simulink model "ModeStEnCtrl6s7s"  (R2018b)
settings: Solver=FixedStepDiscrete  StartTime=0.0  StopTime=10.0  FixedStep=0.01  RelTol=1e-3
undefined symbols (not defined in the file or in its folder): BigFour6sStEnCtrl_Cal, BigFourStEnCtrl_Cal, ComfortMdLStEnCtrl_Cal, ComfortMdRStEnCtrl_Cal, EZE5576sStEnCtrl_Cal, EZE557StEnCtrl_Cal, EZQStEnCtrl_Cal, FirstTrig, INTMLStEnCtrl_Cal, INTMRStEnCtrl_Cal, KeSMSuVehicleModelConfig_Val, LugL6sStEnCtrl_Cal, LugL7sStEnCtrl_Cal, LugR6sStEnCtrl_Cal, LugR7sStEnCtrl_Cal, Md27StEnCtrl_Cal, Md28StEnCtrl_Cal, Md30StEnCtrl_Cal, Md31StEnCtrl_Cal, Md32StEnCtrl_Cal, Md53StEnCtrl_Cal, Md57StEnCtrl_Cal, Md58StEnCtrl_Cal, Md58TrgtPos_Set, Md61StEnCtrl_Cal, Md62StEnCtrl_Cal, RecvR4sStEnCtrl_Cal, VIPL557LTStEnCtrl_Cal, VIPL557StEnCtrl_Cal, VIPLExit557StEnCtrl_Cal, VIPLExit557TrgtPos_Set, VIPR557LTStEnCtrl_Cal, VIPR557StEnCtrl_Cal, VIPRExit557StEnCtrl_Cal, VIPRExit557TrgtPos_Set
libraries: simulink x30
(part 2 of 2)

== system ModeStEnCtrl6s7s/ModeStEnCtrl6s7s_Cal_sys/Subsystem/FamlyLStEnCtrl ==
  note: Delete block
  Enable : EnablePort  StatesWhenEnabling=reset
  Constant : Constant  Value=0  OutDataTypeStr=boolean
  Md62StEnCtrl_Cal : FunctionCaller  FunctionPrototype=Md62StEnCtrl_Cal(FirstTrig)  InputArgumentSpecifications=boolean(true)  OutputArgumentSpecifications=<Enter example>
  Unit Delay : UnitDelay  InitialCondition=1  SampleTime=-1  HasFrameUpgradeWarning=on
  wires:
  Unit Delay/1 -> Md62StEnCtrl_Cal/1
  Constant/1 -> Unit Delay/1

== system ModeStEnCtrl6s7s/ModeStEnCtrl6s7s_Cal_sys/Subsystem/FamlyRStEnCtrl ==
  note: Delete block
  Enable : EnablePort  StatesWhenEnabling=reset
  Constant : Constant  Value=0  OutDataTypeStr=boolean
  Md61StEnCtrl_Cal : FunctionCaller  FunctionPrototype=Md61StEnCtrl_Cal(FirstTrig)  InputArgumentSpecifications=boolean(true)  OutputArgumentSpecifications=<Enter example>
  Unit Delay : UnitDelay  InitialCondition=1  SampleTime=-1  HasFrameUpgradeWarning=on
  wires:
  Unit Delay/1 -> Md61StEnCtrl_Cal/1
  Constant/1 -> Unit Delay/1

== system ModeStEnCtrl6s7s/ModeStEnCtrl6s7s_Cal_sys/Subsystem/INTMLStEnCtrl ==
  note: Delete block
  note: Delete block
  Enable : EnablePort
  INTMLStEnCtrl_Cal : FunctionCaller  FunctionPrototype=INTMLStEnCtrl_Cal()  InputArgumentSpecifications=<Enter example>  OutputArgumentSpecifications=<Enter example>

== system ModeStEnCtrl6s7s/ModeStEnCtrl6s7s_Cal_sys/Subsystem/INTMRStEnCtrl ==
  note: Delete block
  note: Delete block
  Enable : EnablePort
  INTMRStEnCtrl_Cal : FunctionCaller  FunctionPrototype=INTMRStEnCtrl_Cal()  InputArgumentSpecifications=<Enter example>  OutputArgumentSpecifications=<Enter example>

== system ModeStEnCtrl6s7s/ModeStEnCtrl6s7s_Cal_sys/Subsystem/Lug6sLStEnCtrl ==
  note: Delete block
  Enable : EnablePort  StatesWhenEnabling=reset
  LugL6sStEnCtrl_Cal : FunctionCaller  FunctionPrototype=LugL6sStEnCtrl_Cal()  InputArgumentSpecifications=<Enter example>  OutputArgumentSpecifications=<Enter example>

== system ModeStEnCtrl6s7s/ModeStEnCtrl6s7s_Cal_sys/Subsystem/Lug6sRStEnCtrl ==
  note: Delete block
  Enable : EnablePort  StatesWhenEnabling=reset
  LugR6sStEnCtrl_Cal : FunctionCaller  FunctionPrototype=LugR6sStEnCtrl_Cal()  InputArgumentSpecifications=<Enter example>  OutputArgumentSpecifications=<Enter example>

== system ModeStEnCtrl6s7s/ModeStEnCtrl6s7s_Cal_sys/Subsystem/Lug7sLStEnCtrl ==
  Enable : EnablePort  StatesWhenEnabling=reset
  Constant : Constant  Value=0  OutDataTypeStr=boolean
  LugL7sStEnCtrl_Cal : FunctionCaller  FunctionPrototype=LugL7sStEnCtrl_Cal(FirstTrig)  InputArgumentSpecifications=boolean(true)  OutputArgumentSpecifications=<Enter example>
  Unit Delay : UnitDelay  InitialCondition=1  SampleTime=-1  HasFrameUpgradeWarning=on
  wires:
  Unit Delay/1 -> LugL7sStEnCtrl_Cal/1
  Constant/1 -> Unit Delay/1

== system ModeStEnCtrl6s7s/ModeStEnCtrl6s7s_Cal_sys/Subsystem/Lug7sRStEnCtrl ==
  Enable : EnablePort  StatesWhenEnabling=reset
  Constant : Constant  Value=0  OutDataTypeStr=boolean
  LugR7sStEnCtrl_Cal : FunctionCaller  FunctionPrototype=LugR7sStEnCtrl_Cal(FirstTrig)  InputArgumentSpecifications=boolean(true)  OutputArgumentSpecifications=<Enter example>
  Unit Delay : UnitDelay  InitialCondition=1  SampleTime=-1  HasFrameUpgradeWarning=on
  wires:
  Unit Delay/1 -> LugR7sStEnCtrl_Cal/1
  Constant/1 -> Unit Delay/1

== system ModeStEnCtrl6s7s/ModeStEnCtrl6s7s_Cal_sys/Subsystem/Md27StEnCtrl ==
  Enable : EnablePort  StatesWhenEnabling=reset
  Constant : Constant  Value=0  OutDataTypeStr=boolean
  Unit Delay : UnitDelay  InitialCondition=1  SampleTime=-1  HasFrameUpgradeWarning=on
  VIPLExit557StEnCtrl_Cal : FunctionCaller  FunctionPrototype=VIPLExit557StEnCtrl_Cal(FirstTrig)  InputArgumentSpecifications=boolean(true)  OutputArgumentSpecifications=<Enter example>
  wires:
  Constant/1 -> Unit Delay/1
  Unit Delay/1 -> VIPLExit557StEnCtrl_Cal/1

== system ModeStEnCtrl6s7s/ModeStEnCtrl6s7s_Cal_sys/Subsystem/Md27StEnCtrl358  ==
  note: Delete block
  Enable : EnablePort  StatesWhenEnabling=reset
  Md27StEnCtrl_Cal : FunctionCaller  FunctionPrototype=Md27StEnCtrl_Cal()  InputArgumentSpecifications=<Enter example>  OutputArgumentSpecifications=<Enter example>

== system ModeStEnCtrl6s7s/ModeStEnCtrl6s7s_Cal_sys/Subsystem/Md28StEnCtrl ==
  Enable : EnablePort  StatesWhenEnabling=reset
  Constant : Constant  Value=0  OutDataTypeStr=boolean
  Unit Delay : UnitDelay  InitialCondition=1  SampleTime=-1  HasFrameUpgradeWarning=on
  VIPRExit557StEnCtrl_Cal : FunctionCaller  FunctionPrototype=VIPRExit557StEnCtrl_Cal(FirstTrig)  InputArgumentSpecifications=boolean(true)  OutputArgumentSpecifications=<Enter example>
  wires:
  Constant/1 -> Unit Delay/1
  Unit Delay/1 -> VIPRExit557StEnCtrl_Cal/1

== system ModeStEnCtrl6s7s/ModeStEnCtrl6s7s_Cal_sys/Subsystem/Md28StEnCtrl358  ==
  note: Delete block
  Enable : EnablePort  StatesWhenEnabling=reset
  Md28StEnCtrl_Cal : FunctionCaller  FunctionPrototype=Md28StEnCtrl_Cal()  InputArgumentSpecifications=<Enter example>  OutputArgumentSpecifications=<Enter example>

== system ModeStEnCtrl6s7s/ModeStEnCtrl6s7s_Cal_sys/Subsystem/Md30StEnCtrl ==
  Enable : EnablePort  StatesWhenEnabling=reset
  Constant : Constant  Value=0  OutDataTypeStr=boolean
  Md30StEnCtrl_Cal : FunctionCaller  FunctionPrototype=Md30StEnCtrl_Cal(FirstTrig)  InputArgumentSpecifications=boolean(true)  OutputArgumentSpecifications=<Enter example>
  Unit Delay : UnitDelay  InitialCondition=1  SampleTime=-1  HasFrameUpgradeWarning=on
  wires:
  Constant/1 -> Unit Delay/1
  Unit Delay/1 -> Md30StEnCtrl_Cal/1

== system ModeStEnCtrl6s7s/ModeStEnCtrl6s7s_Cal_sys/Subsystem/Md31StEnCtrl ==
  Enable : EnablePort  StatesWhenEnabling=reset
  Constant : Constant  Value=0  OutDataTypeStr=boolean
  Md31StEnCtrl_Cal : FunctionCaller  FunctionPrototype=Md31StEnCtrl_Cal(FirstTrig)  InputArgumentSpecifications=boolean(true)  OutputArgumentSpecifications=<Enter example>
  Unit Delay : UnitDelay  InitialCondition=1  SampleTime=-1  HasFrameUpgradeWarning=on
  wires:
  Constant/1 -> Unit Delay/1
  Unit Delay/1 -> Md31StEnCtrl_Cal/1

== system ModeStEnCtrl6s7s/ModeStEnCtrl6s7s_Cal_sys/Subsystem/Md32StEnCtrl ==
  Enable : EnablePort  StatesWhenEnabling=reset
  Constant : Constant  Value=0  OutDataTypeStr=boolean
  Md32StEnCtrl_Cal : FunctionCaller  FunctionPrototype=Md32StEnCtrl_Cal(FirstTrig)  InputArgumentSpecifications=boolean(true)  OutputArgumentSpecifications=<Enter example>
  Unit Delay : UnitDelay  InitialCondition=1  SampleTime=-1  HasFrameUpgradeWarning=on
  wires:
  Constant/1 -> Unit Delay/1
  Unit Delay/1 -> Md32StEnCtrl_Cal/1

== system ModeStEnCtrl6s7s/ModeStEnCtrl6s7s_Cal_sys/Subsystem/Md53StEnCtrl ==
  Enable : EnablePort  StatesWhenEnabling=reset
  Constant : Constant  Value=0  OutDataTypeStr=boolean
  Md53StEnCtrl_Cal : FunctionCaller  FunctionPrototype=Md53StEnCtrl_Cal(FirstTrig)  InputArgumentSpecifications=boolean(true)  OutputArgumentSpecifications=<Enter example>
  Unit Delay : UnitDelay  InitialCondition=1  SampleTime=-1  HasFrameUpgradeWarning=on
  wires:
  Constant/1 -> Unit Delay/1
  Unit Delay/1 -> Md53StEnCtrl_Cal/1

== system ModeStEnCtrl6s7s/ModeStEnCtrl6s7s_Cal_sys/Subsystem/Md566stEnCtrl ==
  note: Delete block
  Enable : EnablePort  StatesWhenEnabling=reset
  BigFour6sStEnCtrl_Cal : FunctionCaller  FunctionPrototype=BigFour6sStEnCtrl_Cal()  InputArgumentSpecifications=<Enter example>  OutputArgumentSpecifications=<Enter example>

== system ModeStEnCtrl6s7s/ModeStEnCtrl6s7s_Cal_sys/Subsystem/Md56StEnCtrl ==
  note: Delete block
  Enable : EnablePort  StatesWhenEnabling=reset
  BigFourStEnCtrl_Cal : FunctionCaller  FunctionPrototype=BigFourStEnCtrl_Cal(FirstTrig)  InputArgumentSpecifications=boolean(true)  OutputArgumentSpecifications=<Enter example>
  Constant : Constant  Value=0  OutDataTypeStr=boolean
  Unit Delay : UnitDelay  InitialCondition=1  SampleTime=-1  HasFrameUpgradeWarning=on
  wires:
  Constant/1 -> Unit Delay/1
  Unit Delay/1 -> BigFourStEnCtrl_Cal/1

== system ModeStEnCtrl6s7s/ModeStEnCtrl6s7s_Cal_sys/Subsystem/Md57StEnCtrl ==
  note: Delete block
  Enable : EnablePort  StatesWhenEnabling=reset
  Constant : Constant  Value=0  OutDataTypeStr=boolean
  Md57StEnCtrl_Cal : FunctionCaller  FunctionPrototype=Md57StEnCtrl_Cal(FirstTrig)  InputArgumentSpecifications=boolean(true)  OutputArgumentSpecifications=<Enter example>
  Unit Delay : UnitDelay  InitialCondition=1  SampleTime=-1  HasFrameUpgradeWarning=on
  wires:
  Unit Delay/1 -> Md57StEnCtrl_Cal/1
  Constant/1 -> Unit Delay/1

== system ModeStEnCtrl6s7s/ModeStEnCtrl6s7s_Cal_sys/Subsystem/Md58StEnCtrl ==
  note: Delete block
  Enable : EnablePort  StatesWhenEnabling=reset
  Constant : Constant  Value=0  OutDataTypeStr=boolean
  Md58StEnCtrl_Cal : FunctionCaller  FunctionPrototype=Md58StEnCtrl_Cal(FirstTrig)  InputArgumentSpecifications=boolean(true)  OutputArgumentSpecifications=<Enter example>
  Unit Delay : UnitDelay  InitialCondition=1  SampleTime=-1  HasFrameUpgradeWarning=on
  wires:
  Constant/1 -> Unit Delay/1
  Unit Delay/1 -> Md58StEnCtrl_Cal/1

== system ModeStEnCtrl6s7s/ModeStEnCtrl6s7s_Cal_sys/Subsystem/Md58TrgtSet ==
  note: Delete block
  Enable : EnablePort  StatesWhenEnabling=reset
  Md58TrgtPos_Set : FunctionCaller  FunctionPrototype=Md58TrgtPos_Set()  InputArgumentSpecifications=<Enter example>  OutputArgumentSpecifications=<Enter example>

== system ModeStEnCtrl6s7s/ModeStEnCtrl6s7s_Cal_sys/Subsystem/RecvLStEnCtrl ==
  Enable : EnablePort  StatesWhenEnabling=reset
  ComfortMdLStEnCtrl_Cal : FunctionCaller  FunctionPrototype=ComfortMdLStEnCtrl_Cal()

== system ModeStEnCtrl6s7s/ModeStEnCtrl6s7s_Cal_sys/Subsystem/RecvRStEnCtrl ==
  Enable : EnablePort  StatesWhenEnabling=reset
  ComfortMdRStEnCtrl_Cal : FunctionCaller  FunctionPrototype=ComfortMdRStEnCtrl_Cal()

== system ModeStEnCtrl6s7s/ModeStEnCtrl6s7s_Cal_sys/Subsystem/RecvRStEnCtrl1 ==
  Enable : EnablePort  StatesWhenEnabling=reset
  RecvR4sStEnCtrl_Cal : FunctionCaller  FunctionPrototype=RecvR4sStEnCtrl_Cal()

== system ModeStEnCtrl6s7s/ModeStEnCtrl6s7s_Cal_sys/Subsystem/VIPLExitTrgtSet ==
  note: Delete block
  Enable : EnablePort  StatesWhenEnabling=reset
  VIPLExit557TrgtPos_Set : FunctionCaller  FunctionPrototype=VIPLExit557TrgtPos_Set()  InputArgumentSpecifications=<Enter example>  OutputArgumentSpecifications=<Enter example>

== system ModeStEnCtrl6s7s/ModeStEnCtrl6s7s_Cal_sys/Subsystem/VIPLLTStEnCtrl ==
  note: Delete block
  note: Delete block
  note: Delete block
  Enable : EnablePort  StatesWhenEnabling=reset
  VIPL557LTStEnCtrl_Cal : FunctionCaller  FunctionPrototype=VIPL557LTStEnCtrl_Cal()  InputArgumentSpecifications=<Enter example>  OutputArgumentSpecifications=<Enter example>

== system ModeStEnCtrl6s7s/ModeStEnCtrl6s7s_Cal_sys/Subsystem/VIPLStEnCtrl ==
  Enable : EnablePort  StatesWhenEnabling=reset
  Constant : Constant  Value=0  OutDataTypeStr=boolean
  Unit Delay : UnitDelay  InitialCondition=1  SampleTime=-1  HasFrameUpgradeWarning=on
  VIPL557StEnCtrl_Cal : FunctionCaller  FunctionPrototype=VIPL557StEnCtrl_Cal(FirstTrig)  InputArgumentSpecifications=boolean(true)  OutputArgumentSpecifications=<Enter example>
  wires:
  Unit Delay/1 -> VIPL557StEnCtrl_Cal/1
  Constant/1 -> Unit Delay/1

== system ModeStEnCtrl6s7s/ModeStEnCtrl6s7s_Cal_sys/Subsystem/VIPRExitTrgtSet ==
  note: Delete block
  Enable : EnablePort  StatesWhenEnabling=reset
  VIPRExit557TrgtPos_Set : FunctionCaller  FunctionPrototype=VIPRExit557TrgtPos_Set()  InputArgumentSpecifications=<Enter example>  OutputArgumentSpecifications=<Enter example>

== system ModeStEnCtrl6s7s/ModeStEnCtrl6s7s_Cal_sys/Subsystem/VIPRLTStEnCtrl ==
  note: Delete block
  Enable : EnablePort  StatesWhenEnabling=reset
  VIPR557LTStEnCtrl_Cal : FunctionCaller  FunctionPrototype=VIPR557LTStEnCtrl_Cal()  InputArgumentSpecifications=<Enter example>  OutputArgumentSpecifications=<Enter example>

== system ModeStEnCtrl6s7s/ModeStEnCtrl6s7s_Cal_sys/Subsystem/VIPRStEnCtrl ==
  Enable : EnablePort  StatesWhenEnabling=reset
  Constant : Constant  Value=0  OutDataTypeStr=boolean
  Unit Delay : UnitDelay  InitialCondition=1  SampleTime=-1  HasFrameUpgradeWarning=on
  VIPR557StEnCtrl_Cal : FunctionCaller  FunctionPrototype=VIPR557StEnCtrl_Cal(FirstTrig)  InputArgumentSpecifications=boolean(true)  OutputArgumentSpecifications=<Enter example>
  wires:
  Unit Delay/1 -> VIPR557StEnCtrl_Cal/1
  Constant/1 -> Unit Delay/1
